simulink model "lqr_simulink"  (R2024b)
settings: Solver=VariableStepAuto  StartTime=0.0  StopTime=20  RelTol=1e-3
InitFcn:
  | m1 = 250; m2 = 45;
  | k1 = 16000; k2 = 160000;
  | b1 = 1000; b2 = 0;
  | dt = 0.001; T_end = 20; t = 0:dt:T_end;
  | 
  | use_sine = false;
  | if use_sine
  |     freq = 1.27;
  |     w = 0.06 * sin(2*pi*freq*t);
  |     inputType = 'sine';
  | else
  |     w = zeros(size(t));
  |     w(t > 0.5) = 0.1;
  |     inputType = 'step';
  | end
  | 
  | if strcmp(inputType, 'step')
  |     q_body_vel = 1000;
  |     q_integral = 5e7;
  | else
  |     q_body_vel = 1e8;
  |     q_integral = 1e8;
  | end
  | q_body_pos = 250;
  | R = 4e-6;
  | 
  | A = [0, 1, 0, 0; -k1/m1, -b1/m1, k1/m1, b1/m1; 0, 0, 0, 1; k1/m2, b1/m2, -(k1+k2)/m2, -(b1+b2)/m2];
  | B_sim = [0, 0; 1/m1, 0; 0, 0; -1/m2, k2/m2];
  | 
  | % --- FIX START ---
  | C_track = [1 0 0 0]; % Tracks Body Position only
  | D = [0, 0];          % <--- ADD THIS LINE TO FIX THE ERROR
  | % --- FIX END ---
  | 
  | % Note: If you want C to output deflection, use: C = [1 0 -1 0];
  | 
  | % LQR Integral Setup
  | Aa = [A, zeros(4,1); -C_track, 0];
  | Ba = [B_sim(:,1); 0];
  | Qa = diag([q_body_pos, q_body_vel, 100, 100, q_integral]);
  | 
  | K_aug = lqr(Aa, Ba, Qa, R);
  | K_x = K_aug(1:4);
  | K_i = K_aug(5);
  | 
  | RoadData = timeseries(w, t);
  | fprintf('Detected Input: %s | Q_vel: %e | Updated K_i: %f\n', inputType, q_body_vel, K_i);
settings Model: Creator=abdel  LastModifiedBy=abdel

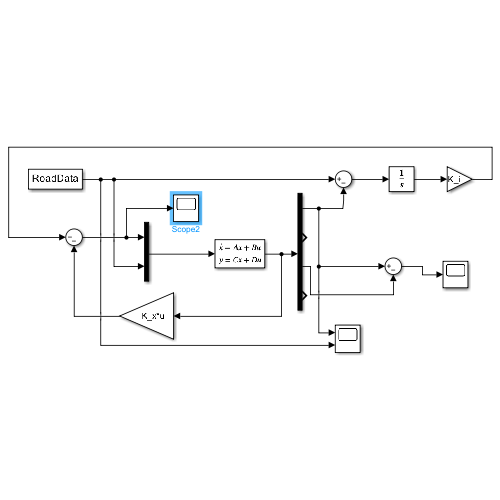
[thumbnail: Simulink's stored preview of the top-level diagram]
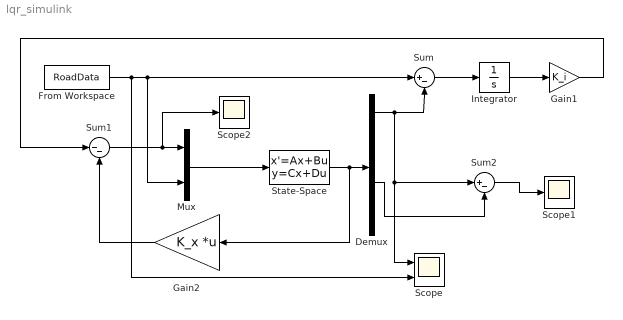
== system lqr_simulink ==
  Demux : Demux
  From Workspace : FromWorkspace  VariableName=RoadData  OutputAfterFinalValue=Setting to zero
  Gain1 : Gain  Gain=K_i
  Gain2 : Gain  Gain=K_x  Multiplication=Matrix(K*u)
  Integrator : Integrator
  Mux : Mux  Inputs=2
  Scope : Scope  NumInputPorts=2
  Scope1 : Scope
  Scope2 : Scope
  State-Space : StateSpace  A=A  B=B_sim  C=eye(4)  D=zeros(4,2)  InitialCondition=[0; 0; 0; 0]
  Sum : Sum  Inputs=|+-
  Sum1 : Sum  Inputs=|--
  Sum2 : Sum  Inputs=|+-
  wires:
  State-Space/1 -> Gain2/1, Demux/1
  From Workspace/1 -> Sum/1, Mux/2, Scope/2
  Sum1/1 -> Scope2/1, Mux/1
  Sum/1 -> Integrator/1
  Mux/1 -> State-Space/1
  Gain2/1 -> Sum1/2
  Demux/1 -> Sum/2, Sum2/1, Scope/1
  Integrator/1 -> Gain1/1
  Gain1/1 -> Sum1/1
  Demux/3 -> Sum2/2
  Sum2/1 -> Scope1/1
